simulink model "ROPOD_Control_WheelsRL_Code_GEN"  (R2020b)
settings: Solver=VariableStepAuto  StartTime=0.0  StopTime=10.0  RelTol=1e-3
values from neighbouring files (symbols this model uses):
  FFtheta_intia = 0    [init_model.m]
  FFxy_mass = 0*80    (= 0)    [init_model.m]
  I_fhz_ddelta_cntr = 0    [init_model.m]
  I_fhz_dtheta_cntr = 0.3    [init_model.m]
  I_fhz_dxdy_cntr = 0.25    [init_model.m]
  K_gain_ddelta_cntr = 0.2    [init_model.m]
  K_gain_dtheta_cntr = 150    [init_model.m]
  K_gain_dxdy_cntr = 200    [init_model.m]
  LL_wp_fhz_ddelta_cntr = 10    [init_model.m]
  LL_wp_fhz_dtheta_cntr = 20    [init_model.m]
  LL_wp_fhz_dxdy_cntr = 20    [init_model.m]
  LL_wz_fhz_ddelta_cntr = 2    [init_model.m]
  LL_wz_fhz_dtheta_cntr = 20    [init_model.m]
  LL_wz_fhz_dxdy_cntr = 20    [init_model.m]
  LPF_fhz_ddelta_cntr = 10    [init_model.m]
  LPF_fhz_ddelta_meas = 50    [init_model.m]
  LPF_fhz_dtheta_cntr = 100    [init_model.m]
  LPF_fhz_dvarphi_meas = 50    [init_model.m]
  LPF_fhz_dxdy_cntr = 100    [init_model.m]
  max_hw_tau = 7.0    (= 7)    [init_model.m]
  max_ropod_acc_theta = 1.6    [init_model.m]
  max_ropod_acc_xy = 2.0    (= 2)    [init_model.m]
  max_ropod_sw_force = 500    [init_model.m]
  max_ropod_sw_tau = 250    [init_model.m]
  max_ropod_vel_theta = 1.6    [init_model.m]
  max_ropod_vel_xy = 2.0    (= 2)    [init_model.m]
  max_sw_current = 10    [init_model.m]
  Nwheels = 4    [Jqwl_numeric_function.m]    (also in S_matrix.m; extract_kinmodel_parameters.m; init_model.m; tau_optimal_dist_vec_fun.m)
  pivot_offs_sws = [3.835 3.465 2.059 0.357]    [init_model.m]
  ropod_kinmodel_pv = struct2array(ropod_kinmodel_param)    [set_ropod_KinModparams.m]
  SW_COM1_ENABLE1 = hex2dec('0001')    [init_model.m]
  SW_COM1_ENABLE2 = hex2dec('0002')    [init_model.m]
  SW_COM1_MODE_TORQUE = bitshift(hex2dec('0000'),2)    [init_model.m]
  SW_COM1_MODE_VELOCITY = bitshift(hex2dec('0002'),2)    [init_model.m]
  SW_COM1_USE_TS = hex2dec('8000')    [init_model.m]
  Tinit = 0*Tslot    [init_model.m]
  Ts = 0.001    [init_model.m]
undefined symbols (not defined in the file or in its folder): AgentNumber, DiscIntNeverNeededParam, flock_FFtheta_friction, flock_FFxy_friction, I_fhz_dtheta_flock_cntr, I_fhz_dvarphi_cntr, I_fhz_dxdy_flock_cntr, K_gain_dtheta_flock_cntr, K_gain_dvarphi_cntr, K_gain_dxdy_flock_cntr, LL_wp_fhz_dtheta_flock_cntr, LL_wp_fhz_dvarphi_cntr, LL_wp_fhz_dxdy_flock_cntr, LL_wz_fhz_dtheta_flock_cntr, LL_wz_fhz_dvarphi_cntr, LL_wz_fhz_dxdy_flock_cntr, LPF_fhz_dtheta_flock_cntr, LPF_fhz_dvarphi_cntr, LPF_fhz_dxdy_flock_cntr, max_flock_acc_theta, max_flock_acc_xy, max_flock_vel_theta, max_flock_vel_xy, Nagents, ropod_position_inflock, sw_tau_2_current, Tsflck
libraries: simulink x62, pid_lib x60, cstblocks x54, dspsigops x24, SOEM_EtherCAT_Lib x5, dspnetwork x4
(part 11 of 11)

== matlab function ROPOD_Control_WheelsRL_Code_GEN/RopodTorqueDistribution/Own Constrainst Calculator ==
  data: enable_local_robot output; ropod_kinmodel_param_vec input; tau_max input; constraints_local_robot output; ena_sw input
function [enable_local_robot, constraints_local_robot ] = calculateConstraints(ropod_kinmodel_param_vec, tau_max, ena_sw)
persistent ena_sw_prev;
persistent tau_max_prev;
persistent constraints_local_robot_internal;
persistent enable_local_robot_internal;

if isempty(ena_sw_prev)
    ena_sw_prev = zeros(size(ena_sw));
    tau_max_prev = 0;
    constraints_local_robot_internal = zeros(8,1);
    enable_local_robot_internal = 0;
end

Nwheels = length(ena_sw);

ena_sw_new = 0;
for i_ena = 1: Nwheels
    if(ena_sw_prev(i_ena)~=ena_sw(i_ena))
        ena_sw_new = 1;
        break;
    end
end

if(   ena_sw_new~=0 ...
   || tau_max_prev ~= tau_max)
    
    [  rW1_1,rW1_2,rW1_3,rW1_4,rW2_1,rW2_2,rW2_3,rW2_4,...
        s_w,...
        d_w, ...
        CW1_1,CW1_2,CW1_3,CW1_4,CW2_1,CW2_2,CW2_3,CW2_4 ...
        ]= extract_kinmodel_parameters(ropod_kinmodel_param_vec);
    
    rw = rW1_1;
    % Conservtaive approach use only forward force of smartwheel, which is
    % the smallest of all directions. In any case forces in other directions
    % last little since the wheels will align in the direction of movement.
    
    Fsw_max = 2*tau_max/rw;
    
    
    CW = [[CW1_1 ; CW2_1], [CW1_2 ; CW2_2], [CW1_3 ; CW2_3], [CW1_4 ; CW2_4]];
    
    
    %% First compute the matrix from v to W_wh
    
    % Gi = zeros([2 3]);
    G = zeros(2*Nwheels,3);
    M = zeros(2*Nwheels,2*Nwheels);
    
    for i=1:Nwheels
        % To obtain pivot velocities in Robot coordinates, add vectors of
        % translations and movement due to angular velocity.
        Gi = [1 0 -CW(2,i);
            0 1  CW(1,i)];
        
        G(2*i-1:2*i,:) = Gi;
        M(2*i-1:2*i,2*i-1:2*i)=diag([ena_sw(i) ena_sw(i)]);
    end
    
    GtS = (M*G)'*eye(8);
    
    if(sum(ena_sw)<2)
        enable_local_robot_internal = 0;
        Fx_max_ropod = 0;
        Fy_max_ropod = 0;
    else
        enable_local_robot_internal = 1;
        % Compute Force at pivots to actuate 1N in x at the ropod. Then scale up.
        Fpiv1Nx = pinv(GtS)*[1 0 0]';
        Fx_max_ropod = Fsw_max/max(abs(Fpiv1Nx));
        Fpiv1Ny = pinv(GtS)*[0 1 0]';
        Fy_max_ropod = Fsw_max/max(abs(Fpiv1Ny));
    end
    
    
    % Eight elements with x,y position of constraint
    constraints_local_robot_internal = ...
        [
        Fx_max_ropod,   0, ...
        0,              Fy_max_ropod , ...
        -Fx_max_ropod,  0, ...
        0,             -Fy_max_ropod  ...
        ]';
    
end

ena_sw_prev = ena_sw;
tau_max_prev = tau_max;

constraints_local_robot = constraints_local_robot_internal;
enable_local_robot = enable_local_robot_internal;



end

== matlab function ROPOD_Control_WheelsRL_Code_GEN/RopodTorqueDistribution_/ROPOD 4SW/ROPOD_4Wheel_sens_own_vel_filter/Glitch removal + LP filter3/Remove_glitches1 ==
  data: vel input; Ts input; encoder input; encoder_out output
function encoder_out  = remove_glitches(vel, Ts, encoder)

persistent last_valid_encoder;
persistent invalid_cnt;

if(isempty(last_valid_encoder))
    last_valid_encoder = encoder;
    invalid_cnt = 0;
end

if abs( (last_valid_encoder-encoder)/Ts ) > 50 % maximum expected velocity rad/sec (2.5 m/s)
    encoder_out = last_valid_encoder + vel*Ts;    
    invalid_cnt = invalid_cnt +1;
else
    encoder_out = encoder;
end

if invalid_cnt>1 
    invalid_cnt = 0;
    encoder_out = encoder;
end

last_valid_encoder = encoder_out;

== matlab function ROPOD_Control_WheelsRL_Code_GEN/RopodTorqueDistribution_/ROPOD 4SW/ROPOD_4Wheel_sens_own_vel_filter/Glitch removal + LP filter4/Remove_glitches1 ==
  data: vel input; Ts input; encoder input; encoder_out output
function encoder_out  = remove_glitches(vel, Ts, encoder)

persistent last_valid_encoder;
persistent invalid_cnt;

if(isempty(last_valid_encoder))
    last_valid_encoder = encoder;
    invalid_cnt = 0;
end

if abs( (last_valid_encoder-encoder)/Ts ) > 50 % maximum expected velocity rad/sec (2.5 m/s)
    encoder_out = last_valid_encoder + vel*Ts;    
    invalid_cnt = invalid_cnt +1;
else
    encoder_out = encoder;
end

if invalid_cnt>1 
    invalid_cnt = 0;
    encoder_out = encoder;
end

last_valid_encoder = encoder_out;

== matlab function ROPOD_Control_WheelsRL_Code_GEN/RopodTorqueDistribution_/ROPOD 4SW/ROPOD_4Wheel_sens_own_vel_filter/Glitch removal + LP filter5/Remove_glitches1 ==
  data: vel input; Ts input; encoder input; encoder_out output
function encoder_out  = remove_glitches(vel, Ts, encoder)

persistent last_valid_encoder;
persistent invalid_cnt;

if(isempty(last_valid_encoder))
    last_valid_encoder = encoder;
    invalid_cnt = 0;
end

if abs( (last_valid_encoder-encoder)/Ts ) > 50 % maximum expected velocity rad/sec (2.5 m/s)
    encoder_out = last_valid_encoder + vel*Ts;    
    invalid_cnt = invalid_cnt +1;
else
    encoder_out = encoder;
end

if invalid_cnt>1 
    invalid_cnt = 0;
    encoder_out = encoder;
end

last_valid_encoder = encoder_out;

== matlab function ROPOD_Control_WheelsRL_Code_GEN/RopodTorqueDistribution_/ROPOD 4SW/ROPOD_4Wheel_sens_own_vel_filter/Glitch removal + LP filter6/Remove_glitches1 ==
  data: vel input; Ts input; encoder input; encoder_out output
function encoder_out  = remove_glitches(vel, Ts, encoder)

persistent last_valid_encoder;
persistent invalid_cnt;

if(isempty(last_valid_encoder))
    last_valid_encoder = encoder;
    invalid_cnt = 0;
end

if abs( (last_valid_encoder-encoder)/Ts ) > 50 % maximum expected velocity rad/sec (2.5 m/s)
    encoder_out = last_valid_encoder + vel*Ts;    
    invalid_cnt = invalid_cnt +1;
else
    encoder_out = encoder;
end

if invalid_cnt>1 
    invalid_cnt = 0;
    encoder_out = encoder;
end

last_valid_encoder = encoder_out;

== matlab function ROPOD_Control_WheelsRL_Code_GEN/RopodTorqueDistribution_/ROPOD 4SW/ROPOD_4Wheel_sens_own_vel_filter/Glitch removal + LP filter7/Remove_glitches1 ==
  data: vel input; Ts input; encoder input; encoder_out output
function encoder_out  = remove_glitches(vel, Ts, encoder)

persistent last_valid_encoder;
persistent invalid_cnt;

if(isempty(last_valid_encoder))
    last_valid_encoder = encoder;
    invalid_cnt = 0;
end

if abs( (last_valid_encoder-encoder)/Ts ) > 50 % maximum expected velocity rad/sec (2.5 m/s)
    encoder_out = last_valid_encoder + vel*Ts;    
    invalid_cnt = invalid_cnt +1;
else
    encoder_out = encoder;
end

if invalid_cnt>1 
    invalid_cnt = 0;
    encoder_out = encoder;
end

last_valid_encoder = encoder_out;

== matlab function ROPOD_Control_WheelsRL_Code_GEN/RopodTorqueDistribution_/ROPOD 4SW/ROPOD_4Wheel_sens_own_vel_filter/Glitch removal + LP filter8/Remove_glitches1 ==
  data: vel input; Ts input; encoder input; encoder_out output
function encoder_out  = remove_glitches(vel, Ts, encoder)

persistent last_valid_encoder;
persistent invalid_cnt;

if(isempty(last_valid_encoder))
    last_valid_encoder = encoder;
    invalid_cnt = 0;
end

if abs( (last_valid_encoder-encoder)/Ts ) > 50 % maximum expected velocity rad/sec (2.5 m/s)
    encoder_out = last_valid_encoder + vel*Ts;    
    invalid_cnt = invalid_cnt +1;
else
    encoder_out = encoder;
end

if invalid_cnt>1 
    invalid_cnt = 0;
    encoder_out = encoder;
end

last_valid_encoder = encoder_out;

== matlab function ROPOD_Control_WheelsRL_Code_GEN/RopodTorqueDistribution_/ROPOD 4SW/ROPOD_4Wheel_sens_own_vel_filter/Glitch removal + LP filter9/Remove_glitches1 ==
  data: vel input; Ts input; encoder input; encoder_out output
function encoder_out  = remove_glitches(vel, Ts, encoder)

persistent last_valid_encoder;
persistent invalid_cnt;

if(isempty(last_valid_encoder))
    last_valid_encoder = encoder;
    invalid_cnt = 0;
end

if abs( (last_valid_encoder-encoder)/Ts ) > 50 % maximum expected velocity rad/sec (2.5 m/s)
    encoder_out = last_valid_encoder + vel*Ts;    
    invalid_cnt = invalid_cnt +1;
else
    encoder_out = encoder;
end

if invalid_cnt>1 
    invalid_cnt = 0;
    encoder_out = encoder;
end

last_valid_encoder = encoder_out;

== matlab function ROPOD_Control_WheelsRL_Code_GEN/RopodTorqueDistribution_/Torque distribution/Gl_matrices ==
  data: ropod_kinmodel_param_vec input; Gl output; delta input; Gtl output; GtSl output
function [Gl, Gtl, GtSl]   = G_matrices( ropod_kinmodel_param_vec, delta)
%ROPOD_JACOBIAN Summary of this function goes here
%   Detailed explanation goes here


Gl    = Gl_matrix_wrapper(ropod_kinmodel_param_vec, delta);
Gtl   = Gl.';
GtSl  = Gtl*S_matrix();
end

== matlab function ROPOD_Control_WheelsRL_Code_GEN/RopodTorqueDistribution_/Torque distribution/platform_forces_2_tau_dist_optimal ==
  data: GtSl input; taubody input; ena_w input; Ttaud output; tau_max input; taubody_sc output
function [Ttaud, taubody_sc]   = Ttaud_optimal_vec( GtSl, taubody, ena_w , tau_max)
%#codegen

[Ttaud, taubody_sc]   = tau_optimal_dist_vec_fun( GtSl, taubody, ena_w, tau_max);

end

== matlab function ROPOD_Control_WheelsRL_Code_GEN/RopodTorqueDistribution_/Torque distribution using pseudoinverse/Gl_matrices ==
  data: ropod_kinmodel_param_vec input; Gl output; delta input; Gtl output; GtSl output
function [Gl, Gtl, GtSl]   = G_matrices( ropod_kinmodel_param_vec, delta)
%ROPOD_JACOBIAN Summary of this function goes here
%   Detailed explanation goes here


Gl    = Gl_matrix_wrapper(ropod_kinmodel_param_vec, delta);
Gtl   = Gl.';
GtSl  = Gtl*S_matrix();
end

== matlab function ROPOD_Control_WheelsRL_Code_GEN/RopodTorqueDistribution/ROPOD 4SW/ROPOD_4Wheel_sens_own_vel_filter/Glitch removal + LP filter/Remove_glitches1 ==
  data: vel input; Ts input; encoder input; encoder_out output
function encoder_out  = remove_glitches(vel, Ts, encoder)

persistent last_valid_encoder;
persistent invalid_cnt;

if(isempty(last_valid_encoder))
    last_valid_encoder = encoder;
    invalid_cnt = 0;
end

if abs( (last_valid_encoder-encoder)/Ts ) > 50 % maximum expected velocity rad/sec (2.5 m/s)
    encoder_out = last_valid_encoder + vel*Ts;    
    invalid_cnt = invalid_cnt +1;
else
    encoder_out = encoder;
end

if invalid_cnt>1 
    invalid_cnt = 0;
    encoder_out = encoder;
end

last_valid_encoder = encoder_out;

== matlab function ROPOD_Control_WheelsRL_Code_GEN/RopodTorqueDistribution_/Torque distribution using pseudoinverse/platform_forces_2_tau_dist_optimal_pseudo_inverse ==
  data: GtSl input; taubody input; ena_w input; varphi_tau output; tau_max input; taubody_sc output
function [varphi_tau, taubody_sc]   = Ttaud_optimal_vec( GtSl, taubody, ena_w , tau_max)
%#codegen

Nwheels = 4;

% Optimization
M = eye(2*Nwheels);
for idx = 1:Nwheels
    M(2*(idx-1)+1,2*(idx-1)+1) = ena_w(idx);
    M(2*(idx-1)+2,2*(idx-1)+2) = ena_w(idx);
end
GM = GtSl*M;

varphi_tau_int = pinv(GM)*taubody;
varphi_tau_int_max = max(abs(varphi_tau_int));
 

if(varphi_tau_int_max > tau_max)
    taubody_sc = tau_max/varphi_tau_int_max;
else
    taubody_sc = 1.0;
end

varphi_tau = taubody_sc*varphi_tau_int;

end

== matlab function ROPOD_Control_WheelsRL_Code_GEN/RopodTorqueDistribution_/wheel flip compensation/MATLAB Function1 ==
  data: tl input; tl_out output; tr input; ropod_kinmodel_param_vec input size=18; tr_out output; kmax input; sc output; Fthr input; tau_max input
function [tl_out,tr_out, sc] = fcn(tl, tr, ropod_kinmodel_param_vec, kmax, Fthr, tau_max)

[  rW1_1,rW1_2,rW1_3,rW1_4,rW2_1,rW2_2,rW2_3,rW2_4,...
    s_w,...
    d_w, ...
    CW1_1,CW1_2,CW1_3,CW1_4,CW2_1,CW2_2,CW2_3,CW2_4 ...
    ]= extract_kinmodel_parameters(ropod_kinmodel_param_vec);

Fxi = (tl/rW1_1+tr/rW1_2);
Fyi = (tr/rW1_2-tl/rW1_1)*(d_w/(2*s_w));
theta = atan2(Fyi,Fxi);

Fsize = abs(Fyi);
if Fsize> Fthr
   sc = (1+(kmax-1)*abs( sin(theta)) );
else
    sc = 1;
end

avg_t = (tr+tl)/2;
diff_t = (tr-tl)/2;
tl_out = avg_t-sc*diff_t;
tr_out = avg_t+sc*diff_t;

if(abs(tl_out)>tau_max && abs(tl_out)>abs(tr_out))
    sc = tau_max/abs(tl_out);
    tl_out = sc*tl_out;
    tr_out = sc*tr_out;
end

if(abs(tr_out)>tau_max && abs(tr_out)>abs(tl_out))
    sc = tau_max/abs(tr_out);
    tl_out = sc*tl_out;
    tr_out = sc*tr_out;
end

== matlab function ROPOD_Control_WheelsRL_Code_GEN/RopodTorqueDistribution_/wheel flip compensation/MATLAB Function2 ==
  data: tl input; tl_out output; tr input; ropod_kinmodel_param_vec input size=18; tr_out output; kmax input; sc output; Fthr input; tau_max input
function [tl_out,tr_out, sc] = fcn(tl, tr, ropod_kinmodel_param_vec, kmax, Fthr, tau_max)

[  rW1_1,rW1_2,rW1_3,rW1_4,rW2_1,rW2_2,rW2_3,rW2_4,...
    s_w,...
    d_w, ...
    CW1_1,CW1_2,CW1_3,CW1_4,CW2_1,CW2_2,CW2_3,CW2_4 ...
    ]= extract_kinmodel_parameters(ropod_kinmodel_param_vec);

Fxi = (tl/rW1_1+tr/rW1_2);
Fyi = (tr/rW1_2-tl/rW1_1)*(d_w/(2*s_w));
theta = atan2(Fyi,Fxi);

Fsize = abs(Fyi);
if Fsize> Fthr
   sc = (1+(kmax-1)*abs( sin(theta)) );
else
    sc = 1;
end

avg_t = (tr+tl)/2;
diff_t = (tr-tl)/2;
tl_out = avg_t-sc*diff_t;
tr_out = avg_t+sc*diff_t;

if(abs(tl_out)>tau_max && abs(tl_out)>abs(tr_out))
    sc = tau_max/abs(tl_out);
    tl_out = sc*tl_out;
    tr_out = sc*tr_out;
end

if(abs(tr_out)>tau_max && abs(tr_out)>abs(tl_out))
    sc = tau_max/abs(tr_out);
    tl_out = sc*tl_out;
    tr_out = sc*tr_out;
end

== matlab function ROPOD_Control_WheelsRL_Code_GEN/RopodTorqueDistribution_/wheel flip compensation/MATLAB Function3 ==
  data: tl input; tl_out output; tr input; ropod_kinmodel_param_vec input size=18; tr_out output; kmax input; sc output; Fthr input; tau_max input
function [tl_out,tr_out, sc] = fcn(tl, tr, ropod_kinmodel_param_vec, kmax, Fthr, tau_max)

[  rW1_1,rW1_2,rW1_3,rW1_4,rW2_1,rW2_2,rW2_3,rW2_4,...
    s_w,...
    d_w, ...
    CW1_1,CW1_2,CW1_3,CW1_4,CW2_1,CW2_2,CW2_3,CW2_4 ...
    ]= extract_kinmodel_parameters(ropod_kinmodel_param_vec);

Fxi = (tl/rW1_1+tr/rW1_2);
Fyi = (tr/rW1_2-tl/rW1_1)*(d_w/(2*s_w));
theta = atan2(Fyi,Fxi);

Fsize = abs(Fyi);
if Fsize> Fthr
   sc = (1+(kmax-1)*abs( sin(theta)) );
else
    sc = 1;
end

avg_t = (tr+tl)/2;
diff_t = (tr-tl)/2;
tl_out = avg_t-sc*diff_t;
tr_out = avg_t+sc*diff_t;

if(abs(tl_out)>tau_max && abs(tl_out)>abs(tr_out))
    sc = tau_max/abs(tl_out);
    tl_out = sc*tl_out;
    tr_out = sc*tr_out;
end

if(abs(tr_out)>tau_max && abs(tr_out)>abs(tl_out))
    sc = tau_max/abs(tr_out);
    tl_out = sc*tl_out;
    tr_out = sc*tr_out;
end

== matlab function ROPOD_Control_WheelsRL_Code_GEN/RopodTorqueDistribution_/wheel flip compensation/MATLAB Function4 ==
  data: tl input; tl_out output; tr input; ropod_kinmodel_param_vec input size=18; tr_out output; kmax input; sc output; Fthr input; tau_max input
function [tl_out,tr_out, sc] = fcn(tl, tr, ropod_kinmodel_param_vec, kmax, Fthr, tau_max)

[  rW1_1,rW1_2,rW1_3,rW1_4,rW2_1,rW2_2,rW2_3,rW2_4,...
    s_w,...
    d_w, ...
    CW1_1,CW1_2,CW1_3,CW1_4,CW2_1,CW2_2,CW2_3,CW2_4 ...
    ]= extract_kinmodel_parameters(ropod_kinmodel_param_vec);

Fxi = (tl/rW1_1+tr/rW1_2);
Fyi = (tr/rW1_2-tl/rW1_1)*(d_w/(2*s_w));
theta = atan2(Fyi,Fxi);

Fsize = abs(Fyi);
if Fsize> Fthr
   sc = (1+(kmax-1)*abs( sin(theta)) );
else
    sc = 1;
end

avg_t = (tr+tl)/2;
diff_t = (tr-tl)/2;
tl_out = avg_t-sc*diff_t;
tr_out = avg_t+sc*diff_t;

if(abs(tl_out)>tau_max && abs(tl_out)>abs(tr_out))
    sc = tau_max/abs(tl_out);
    tl_out = sc*tl_out;
    tr_out = sc*tr_out;
end

if(abs(tr_out)>tau_max && abs(tr_out)>abs(tl_out))
    sc = tau_max/abs(tr_out);
    tl_out = sc*tl_out;
    tr_out = sc*tr_out;
end

== matlab function ROPOD_Control_WheelsRL_Code_GEN/RopodProcessWheelSensorData_/Odometry and Measurement model 4SW/Jqwl_numeric ==
  data: ropod_kinmodel_param_vec input; v output; delta input; dvarphi input; ena_w input
function v = Jqwl_numeric_wrapper(ropod_kinmodel_param_vec,  delta, dvarphi, ena_w)

v = Jqwl_numeric_function(ropod_kinmodel_param_vec, delta, dvarphi, ena_w);

end

== matlab function ROPOD_Control_WheelsRL_Code_GEN/RopodProcessWheelSensorData_/Odometry and Measurement model 4SW/pos_rot_matrix ==
  data: dqr_loc input; theta_odom input; dqr_glb output
function dqr_glb   = zrot(dqr_loc, theta_odom)
%ROPOD_JACOBIAN Summary of this function goes here
%   Detailed explanation goes here


dqr_glb = [  cos(theta_odom) -sin(theta_odom) 0; 
            sin(theta_odom)  cos(theta_odom) 0;
                    0             0  1]*dqr_loc;
end

== matlab function ROPOD_Control_WheelsRL_Code_GEN/RopodTorqueDistribution/ROPOD 4SW/ROPOD_4Wheel_sens_own_vel_filter/Glitch removal + LP filter1/Remove_glitches1 ==
  data: vel input; Ts input; encoder input; encoder_out output
function encoder_out  = remove_glitches(vel, Ts, encoder)

persistent last_valid_encoder;
persistent invalid_cnt;

if(isempty(last_valid_encoder))
    last_valid_encoder = encoder;
    invalid_cnt = 0;
end

if abs( (last_valid_encoder-encoder)/Ts ) > 50 % maximum expected velocity rad/sec (2.5 m/s)
    encoder_out = last_valid_encoder + vel*Ts;    
    invalid_cnt = invalid_cnt +1;
else
    encoder_out = encoder;
end

if invalid_cnt>1 
    invalid_cnt = 0;
    encoder_out = encoder;
end

last_valid_encoder = encoder_out;

== matlab function ROPOD_Control_WheelsRL_Code_GEN/RopodProcessWheelSensorData/Odometry and Measurement model 4SW/Jqwl_numeric ==
  data: ropod_kinmodel_param_vec input; v output; delta input; dvarphi input; ena_w input
function v = Jqwl_numeric_wrapper(ropod_kinmodel_param_vec,  delta, dvarphi, ena_w)

v = Jqwl_numeric_function(ropod_kinmodel_param_vec, delta, dvarphi, ena_w);

end

== matlab function ROPOD_Control_WheelsRL_Code_GEN/RopodProcessWheelSensorData/Odometry and Measurement model 4SW/pos_rot_matrix ==
  data: dqr_loc input; theta_odom input; dqr_glb output
function dqr_glb   = zrot(dqr_loc, theta_odom)
%ROPOD_JACOBIAN Summary of this function goes here
%   Detailed explanation goes here


dqr_glb = [  cos(theta_odom) -sin(theta_odom) 0; 
            sin(theta_odom)  cos(theta_odom) 0;
                    0             0  1]*dqr_loc;
end

== matlab function ROPOD_Control_WheelsRL_Code_GEN/RopodTorqueDistribution/ROPOD 4SW/ROPOD_4Wheel_sens_own_vel_filter/Glitch removal + LP filter2/Remove_glitches1 ==
  data: vel input; Ts input; encoder input; encoder_out output
function encoder_out  = remove_glitches(vel, Ts, encoder)

persistent last_valid_encoder;
persistent invalid_cnt;

if(isempty(last_valid_encoder))
    last_valid_encoder = encoder;
    invalid_cnt = 0;
end

if abs( (last_valid_encoder-encoder)/Ts ) > 50 % maximum expected velocity rad/sec (2.5 m/s)
    encoder_out = last_valid_encoder + vel*Ts;    
    invalid_cnt = invalid_cnt +1;
else
    encoder_out = encoder;
end

if invalid_cnt>1 
    invalid_cnt = 0;
    encoder_out = encoder;
end

last_valid_encoder = encoder_out;

== matlab function ROPOD_Control_WheelsRL_Code_GEN/RopodTorqueDistribution/ROPOD 4SW/ROPOD_4Wheel_sens_own_vel_filter/Glitch removal + LP filter3/Remove_glitches1 ==
  data: vel input; Ts input; encoder input; encoder_out output
function encoder_out  = remove_glitches(vel, Ts, encoder)

persistent last_valid_encoder;
persistent invalid_cnt;

if(isempty(last_valid_encoder))
    last_valid_encoder = encoder;
    invalid_cnt = 0;
end

if abs( (last_valid_encoder-encoder)/Ts ) > 50 % maximum expected velocity rad/sec (2.5 m/s)
    encoder_out = last_valid_encoder + vel*Ts;    
    invalid_cnt = invalid_cnt +1;
else
    encoder_out = encoder;
end

if invalid_cnt>1 
    invalid_cnt = 0;
    encoder_out = encoder;
end

last_valid_encoder = encoder_out;
